simulink model "ensaio_torque_velocidade"  (R2015a)
settings: Solver=ode45  StartTime=0.0  StopTime=6.0  RelTol=1e-3
values from neighbouring files (symbols this model uses):
  Ts = 2e-05    [script_torque_velocidade.m]
libraries: powerlib x5, powerlib_meascontrol x3, simulink x1
settings Model: Creator=range  LastModifiedBy=range

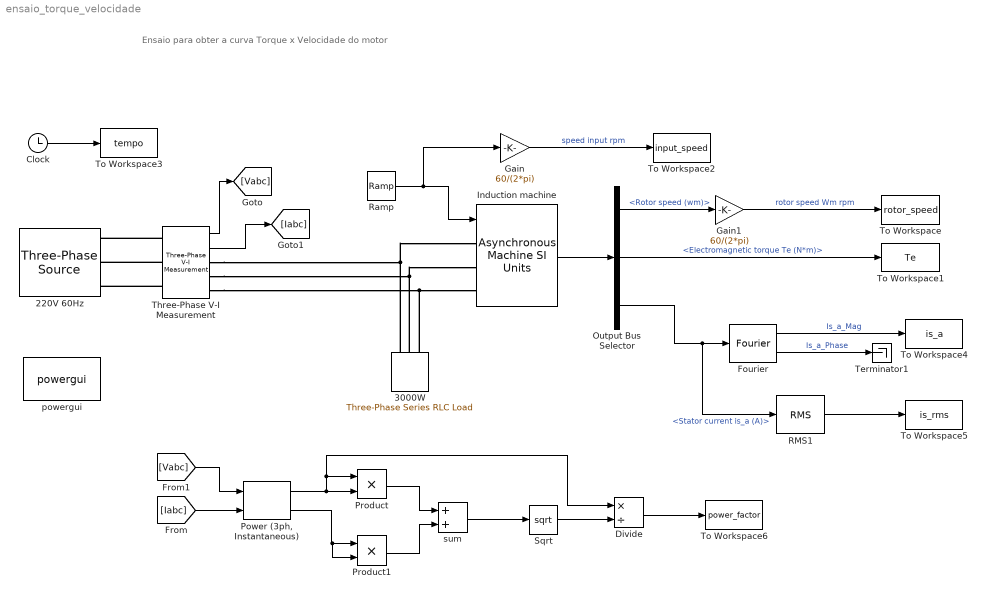
== system ensaio_torque_velocidade ==
  note: Ensaio para obter a curva Torque x Velocidade do motor
  220V 60Hz : powerlib/Electrical Sources/Three-Phase Source  Voltage=220  PhaseAngle=0  Frequency=60  InternalConnection=Yg  SpecifyImpedance=off  Resistance=0.5  Inductance=0.1e-3  ShortCircuitLevel=0  BaseVoltage=0  XRratio=0  BusType=swing  Pref=0  Qref=0  Qmin=-inf  Qmax=inf
  3000W : powerlib/Elements/Three-Phase Series RLC Load  LConnTagsString=A|B|C  Configuration=Y (grounded)  NominalVoltage=220  NominalFrequency=60  ActivePower=30000  InductivePower=0  CapacitivePower=0  Measurements=None  LoadType=constant Z
  Clock : Clock
  Divide : Product  Inputs=*/
  Fourier : powerlib_meascontrol/Measurements/Fourier  Freq=60  n=1  InInit=[0, 0]  Ts=Ts
  Gain : Gain  Gain=60/(2*pi)
  Gain1 : Gain  Gain=60/(2*pi)
  Induction machine : powerlib/Machines/Asynchronous Machine SI Units  RotorType=Squirrel-cage  PresetModel=No  MechanicalLoad=Speed w  ShowDetailedParameters=on  ReferenceFrame=Stationary  Units=SI  MeasurementBus=off  NominalParameters=[2238,220,60]  Stator=[0.435,0.002]  Rotor=[0.816,0.002]  Cage1=[ 0.022 0.226/377]  Cage2=[ 0.022 0.226/377]  Lm=69.31e-3  Mechanical=[0.089,0.005,2]  PolePairs=2  InitialConditions=[1,0,0,0,0,0,0,0]  SimulateSaturation=off  Saturation=[0 0;0 0]  LoadFlowParameters=0  TsPowergui=0  TsBlock=-1  IterativeModel=Trapezoidal non iterative  Pmec=0
  Output Bus Selector : BusSelector  OutputSignals=Mechanical.Rotor speed (wm),Mechanical.Electromagnetic torque Te (N*m),Stator measurements.Stator current is_a (A)
  "Power (3ph, Instantaneous)" : powerlib_meascontrol/Measurements/Power (3ph, Instantaneous)
  Product : Product
  Product1 : Product
  RMS1 : powerlib_meascontrol/Measurements/RMS  TrueRMS=on  Freq=60  RMSInit=0  Ts=Ts
  Ramp : simulink/Sources/Ramp  slope=37.7  start=0  X0=0
  Sqrt : Sqrt  SaturateOnIntegerOverflow=on
  Terminator1 : Terminator
  Three-Phase V-I Measurement : powerlib/Measurements/Three-Phase V-I Measurement  VoltageMeasurement=phase-to-ground  SetLabelV=off  LabelV=Vabc  Vpu=off  VpuLL=off  CurrentMeasurement=yes  SetLabelI=off  LabelI=Iabc  Ipu=off  Pbase=100e6  Vbase=500e3  OutputType=Complex  PhasorSimulation=off  PSBequivalent=0
  To Workspace : ToWorkspace  VariableName=rotor_speed  SampleTime=Ts
  To Workspace1 : ToWorkspace  VariableName=Te  SampleTime=Ts
  To Workspace2 : ToWorkspace  VariableName=input_speed  SampleTime=Ts
  To Workspace3 : ToWorkspace  VariableName=tempo  SampleTime=Ts
  To Workspace4 : ToWorkspace  VariableName=is_a  SampleTime=Ts
  To Workspace5 : ToWorkspace  VariableName=is_rms  SampleTime=Ts
  To Workspace6 : ToWorkspace  VariableName=power_factor  SampleTime=Ts
  powergui : powerlib/powergui  Priority=2  SimulationMode=Discrete  SolverType=Tustin/Backward Euler (TBE)  SampleTime=Ts  frequency=60  SPID=off  DisableSnubberDevices=on  DisableRonSwitches=off  DisableVfSwitches=off  SwTol=0  DisplayEquations=off  Interpol=off  methode=off  Ts=0  FunctionMessages=off  echomessages=off  HookPort=off  EnableUseOfTLC=off  x0status=blocks  frequencyindice=60  Pbase=100e6  ErrMax=1e-4  Iterations=50  UnitsV=kV  UnitsW=MW  buscounter=0  RestoreLinks=warning  ResistiveCurrentMeasurement=off  Frange=[0:2:500]  Ylog=off  Xlog=on  ShowGrid=off  save=off  variable=ZData  structure=0  ZoomFFT=on  StartTime=0.0  cycles=1  DisplayStyle=1  fundamental=60  FreqAxis=off  MaxFrequency=1000  frequencyindicesteady=1  RmsSteady=1  display=off
  "sum " : Sum
  wires:
  Induction machine/1 -> Output Bus Selector/1
  Ramp/1 -> Gain/1, Induction machine/1
  Gain/1 -> To Workspace2/1  "speed input rpm"
  Output Bus Selector/1 -> Gain1/1  "<Rotor speed (wm)>"
  Gain1/1 -> To Workspace/1  "rotor speed Wm rpm"
  Output Bus Selector/2 -> To Workspace1/1  "<Electromagnetic torque Te (N*m)>"
  Clock/1 -> To Workspace3/1
  Output Bus Selector/3 -> RMS1/1, Fourier/1  "<Stator current is_a (A)>"
  Fourier/2 -> Terminator1/1  "Is_a_Phase"
  Fourier/1 -> To Workspace4/1  "Is_a_Mag"
  RMS1/1 -> To Workspace5/1
  Three-Phase V-I Measurement/1 -> [Vabc]
  Three-Phase V-I Measurement/2 -> [Iabc]
  [Iabc] -> "Power (3ph, Instantaneous)"/2
  [Vabc] -> "Power (3ph, Instantaneous)"/1
  "Power (3ph, Instantaneous)"/2 -> Product1/2, Product1/1
  "Power (3ph, Instantaneous)"/1 -> Divide/1, Product/1, Product/2
  Product/1 -> "sum "/1
  Product1/1 -> "sum "/2
  "sum "/1 -> Sqrt/1
  Sqrt/1 -> Divide/2
  Divide/1 -> To Workspace6/1
  connections:
  3000W/LConn1 -- Three-Phase V-I Measurement/RConn1 -- Induction machine/LConn1
  3000W/LConn2 -- Three-Phase V-I Measurement/RConn2 -- Induction machine/LConn2
  3000W/LConn3 -- Three-Phase V-I Measurement/RConn3 -- Induction machine/LConn3
  Three-Phase V-I Measurement/LConn3 -- 220V 60Hz/RConn3
  Three-Phase V-I Measurement/LConn2 -- 220V 60Hz/RConn2
  Three-Phase V-I Measurement/LConn1 -- 220V 60Hz/RConn1
